simulink model "Phase2_Section3_State_Feedback"  (R2021b)
settings: Solver=VariableStepAuto  StartTime=0.0  StopTime=50  RelTol=1e-3
values from neighbouring files (symbols this model uses):
  A = [0 1 0; 244.86 -0.094 -26.29; 0 0 -250]    [Phase2_Section1.m]    (also in Phase2_Section2.m; Phase2_Section3.m; Phase2_Section4.m; Phase2_Section5.m)
  B = [0; 0; 5]    [Phase2_Section1.m]    (also in Phase2_Section2.m; Phase2_Section3.m; Phase2_Section4.m; Phase2_Section5.m)
  C = [1 0 0]    [Phase2_Section1.m]    (also in Phase2_Section2.m; Phase2_Section3.m; Phase2_Section4.m; Phase2_Section5.m)
  K1 = place(A, B, p_fast)    [Phase2_Section1.m]    (also in Phase2_Section2.m; Phase2_Section3.m; Phase2_Section4.m = place(A, B, [-4 -2 -3]); Phase2_Section5.m = place(A, B, [-4 -2 -3]))
settings Model: Creator=USER  LastModifiedBy=odeut

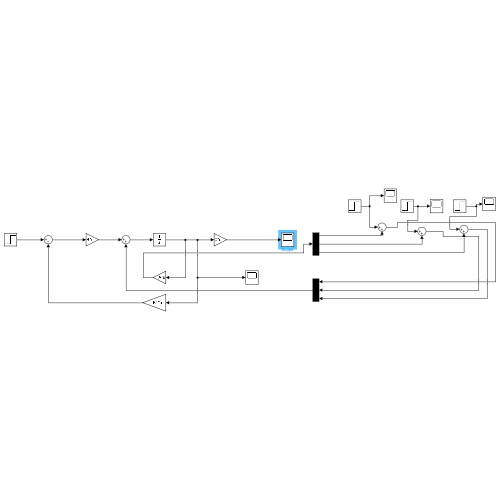
[thumbnail: Simulink's stored preview of the top-level diagram]
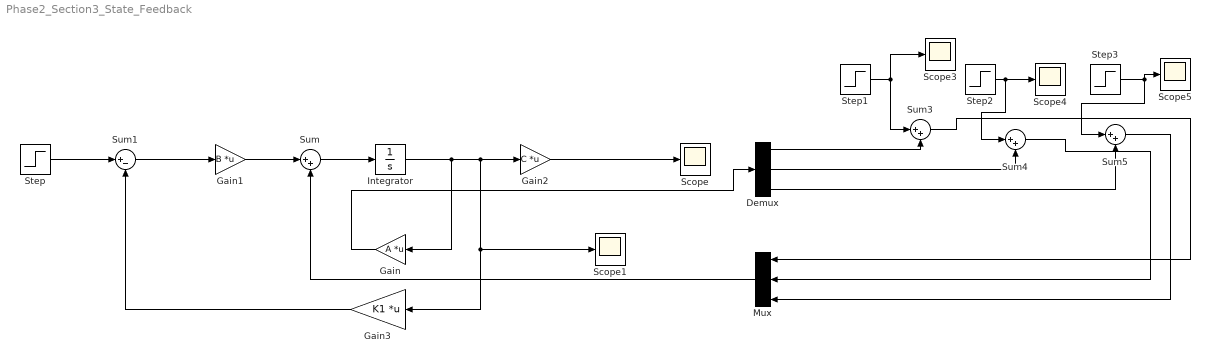
== system Phase2_Section3_State_Feedback ==
  Demux : Demux  Outputs=3
  Gain : Gain  Gain=A  Multiplication=Matrix(K*u)
  Gain1 : Gain  Gain=B  Multiplication=Matrix(K*u)
  Gain2 : Gain  Gain=C  Multiplication=Matrix(K*u)
  Gain3 : Gain  Gain=K1  Multiplication=Matrix(K*u)
  Integrator : Integrator
  Mux : Mux  Inputs=3
  Scope{,1,3..5} (5 alike) : Scope
  Step : Step  SampleTime=0
  Step1 : Step  Time=4  SampleTime=0
  Step2 : Step  Time=4  SampleTime=0
  Step3 : Step  Time=4  SampleTime=0
  Sum{,3..5} (4 alike) : Sum  Inputs=|++
  Sum1 : Sum  Inputs=|+-
  wires:
  Step2/1 -> Sum4/1, Scope4/1
  Sum4/1 -> Mux/2
  Demux/3 -> Sum5/2
  Step3/1 -> Sum5/1, Scope5/1
  Sum5/1 -> Mux/3
  Sum3/1 -> Mux/1
  Demux/2 -> Sum4/2
  Step1/1 -> Sum3/1, Scope3/1
  Demux/1 -> Sum3/2
  Gain1/1 -> Sum/1
  Sum1/1 -> Gain1/1
  Step/1 -> Sum1/1
  Gain2/1 -> Scope/1
  Gain3/1 -> Sum1/2
  Integrator/1 -> Gain/1, Scope1/1, Gain3/1, Gain2/1
  Sum/1 -> Integrator/1
  Gain/1 -> Demux/1
  Mux/1 -> Sum/2
